simulink model "lrq"  (R2021b)
settings: Solver=VariableStepAuto  StartTime=0.0  StopTime=10  RelTol=1e-3
settings Model: Creator=84232  LastModifiedBy=84232

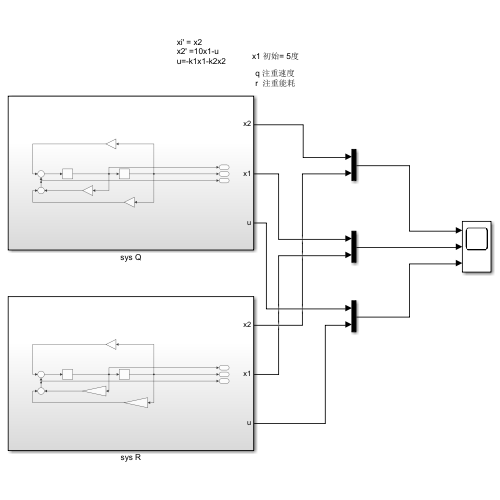
[thumbnail: Simulink's stored preview of the top-level diagram]
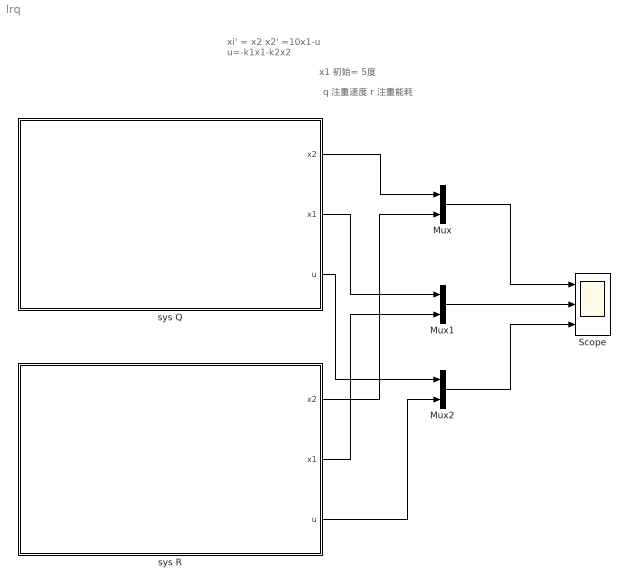
== system lrq ==
  note: q 注重速度
      | r  注重能耗
  note: x1 初始= 5度
  note: xi' = x2
      | x2' =10x1-u
      | u=-k1x1-k2x2
  Mux : Mux  Inputs=2
  Mux1 : Mux  Inputs=2
  Mux2 : Mux  Inputs=2
  Scope : Scope  NumInputPorts=3
  sys Q : Subsystem
  sys R : Subsystem
  wires:
  sys Q/1(x2) -> Mux/1
  sys R/1(x2) -> Mux/2
  sys Q/2(x1) -> Mux1/1
  sys R/2(x1) -> Mux1/2
  sys R/3(u) -> Mux2/2
  sys Q/3(u) -> Mux2/1
  Mux1/1 -> Scope/2
  Mux/1 -> Scope/1
  Mux2/1 -> Scope/3

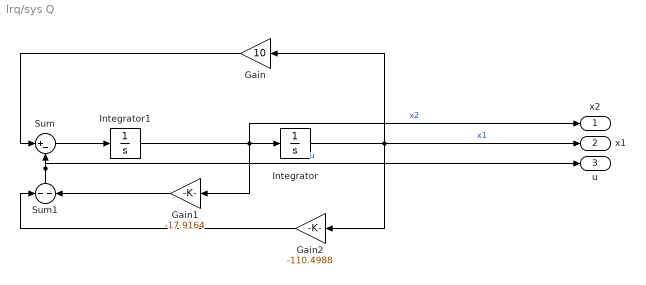
== system lrq/sys Q ==
  Gain : Gain  Gain=10
  Gain1 : Gain  Gain=-17.9164
  Gain2 : Gain  Gain=-110.4988
  Integrator : Integrator  InitialCondition=5
  Integrator1 : Integrator
  Sum : Sum  Inputs=|+-
  Sum1 : Sum  Inputs=--
  x2 : Outport
  x1 : Outport  Port=2
  u : Outport  Port=3
  wires:
  Gain/1 -> Sum/1
  Integrator1/1 -> x2/1, Gain1/1, Integrator/1  "x2"
  Sum1/1 -> u/1, Sum/2  "u"
  Integrator/1 -> x1/1, Gain/1, Gain2/1  "x1"
  Gain1/1 -> Sum1/2
  Gain2/1 -> Sum1/1
  Sum/1 -> Integrator1/1

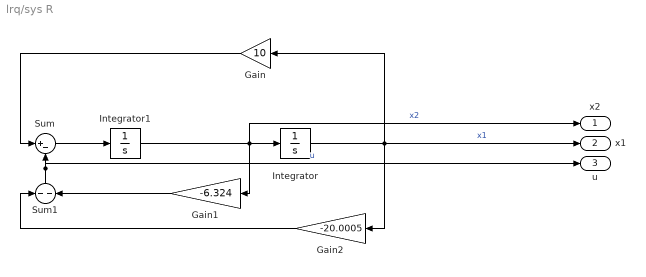
== system lrq/sys R ==
  Gain : Gain  Gain=10
  Gain1 : Gain  Gain=-6.324
  Gain2 : Gain  Gain=-20.0005
  Integrator : Integrator  InitialCondition=5
  Integrator1 : Integrator
  Sum : Sum  Inputs=|+-
  Sum1 : Sum  Inputs=--
  x2 : Outport
  x1 : Outport  Port=2
  u : Outport  Port=3
  wires:
  Gain/1 -> Sum/1
  Integrator1/1 -> x2/1, Gain1/1, Integrator/1  "x2"
  Sum1/1 -> u/1, Sum/2  "u"
  Integrator/1 -> x1/1, Gain/1, Gain2/1  "x1"
  Gain1/1 -> Sum1/2
  Gain2/1 -> Sum1/1
  Sum/1 -> Integrator1/1
